simulink library "lib_GenTools_LogisticFun"  (R2015a)
settings: Solver=ode45  StartTime=0.0  StopTime=10.0  RelTol=1e-3
settings Model: Creator=jlkratz  LastModifiedBy=jlkratz

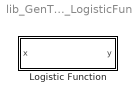
== system lib_GenTools_LogisticFun ==
  Logistic Function : Subsystem  mask(TSAT: Logistic Function){Lo_M=1, Lf_M=2, kCalc_M=on, k_M=1, xoCalc_M=off, xo_M=0, xL_M=-1, xR_M=1}
      mask prompts: Lo_M "Lo_M - value of the fuction at the left asymptote"; Lf_M "Lf_M - value of the fucntion at the right asymptote"; kCalc_M "kCalc_M - Checked - Calculate k in initialization, Unchecked - spedfy k as a parameter"; k_M "k_M - Logistic function slope"; xoCalc_M "xoCalc_M - Checked - Calculate xo in initialization, Unchecked - spedfy xo as a parameter"; xo_M "xo_M - Function shift in the x-direction"; xL_M "xL_M - x locatioin where y is within 1% of Lo_M"; xR_M "xR_M - x location where y is within 1% of Lf_M"
      mask help:
      | This block defines logistic function:
      |
      | y = (Lf - Lo)/(1 + exp(-k*(x-xo))) + Lo
      |
      | where x is the independent variable.
      mask init:
      | if xoCalc_M == 1
      |     xo_I = 0.5*(xR_M + xL_M);
      | else
      |     xo_I = xo_M;
      | end
      | 
      | if kCalc_M == 1
      |     k_I = -log(99)/(xL_M-xo_I);
      | else 
      |     k_I = k_M;
      | end
      mask Help: web(which('GenTools_TSAT_LogisticFun.html'),'-helpbrowser')
      mask Callback kCalc_M:
      | %k_M
      | MSK_SEC_Enables_TSAT('kCalc_M',4,'dis');
      | 
      | %xL_M & xR_M
      | if length(get_param(gcb,'xoCalc_M')) == 2
      |     %do nothing
      | elseif length(get_param(gcb,'kCalc_M')) == 2
      |     MSK_SEC_Enables2_TSAT('kCalc_M',7,'en');
      |     MSK_SEC_Enables2_TSAT('kCalc_M',8,'en');
      | else
      |     MSK_SEC_Enables2_TSAT('kCalc_M',7,'dis');
      |     MSK_SEC_Enables2_TSAT('kCalc_M',8,'dis');
      | end
      mask Callback xoCalc_M:
      | %xo_M
      | MSK_SEC_Enables_TSAT('xoCalc_M',6,'dis');
      | 
      | %xL_M & xR_M
      | if length(get_param(gcb,'kCalc_M')) == 2
      |     %do nothing
      | elseif length(get_param(gcb,'xoCalc_M')) == 2
      |     MSK_SEC_Enables2_TSAT('xoCalc_M',7,'en');
      |     MSK_SEC_Enables2_TSAT('xoCalc_M',8,'en');
      | else
      |     MSK_SEC_Enables2_TSAT('xoCalc_M',7,'dis');
      |     MSK_SEC_Enables2_TSAT('xoCalc_M',8,'dis');
      | end

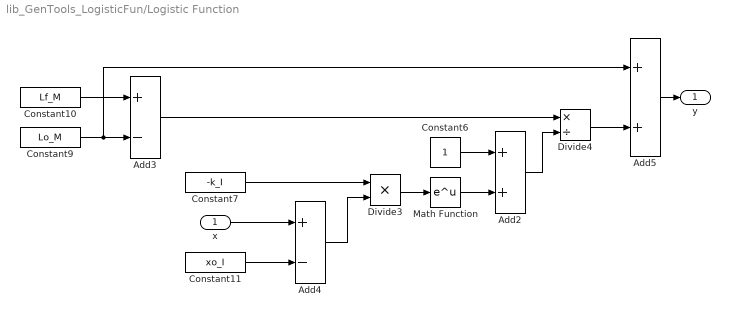
== system lib_GenTools_LogisticFun/Logistic Function ==
  x : Inport
  Add2 : Sum
  Add3 : Sum  Inputs=+-
  Add4 : Sum  Inputs=+-
  Add5 : Sum
  Constant10 : Constant  Value=Lf_M
  Constant11 : Constant  Value=xo_I
  Constant6 : Constant
  Constant7 : Constant  Value=-k_I
  Constant9 : Constant  Value=Lo_M
  Divide3 : Product  Inputs=**
  Divide4 : Product  Inputs=*/
  Math Function : Math  SaturateOnIntegerOverflow=on
  y : Outport
  wires:
  Math Function/1 -> Add2/2
  Divide3/1 -> Math Function/1
  Constant7/1 -> Divide3/1
  Add3/1 -> Divide4/1
  Constant6/1 -> Add2/1
  Divide4/1 -> Add5/2
  x/1 -> Add4/1
  Constant9/1 -> Add3/2, Add5/1
  Add4/1 -> Divide3/2
  Constant11/1 -> Add4/2
  Constant10/1 -> Add3/1
  Add5/1 -> y/1
  Add2/1 -> Divide4/2
